simulink model "model_prawego_zbiornika"  (R2023b)
settings: Solver=ode1  StartTime=0.0  StopTime=200  FixedStep=0.02  RelTol=1e-3
undefined symbols (not defined in the file or in its folder): DiscIntNeverNeededParam
libraries: slctrl_adaptive x1, fuzblock x1, slpidlib x1, simulink x1
settings Model: Creator=kerif  LastModifiedBy=kerif
settings ConfigComp: PLC_TargetIDE=codesys35  PLC_MultiTBSigbuilderTimeRange=off  PLC_FoldFBCallOutputVar=off  PLC_RemoveUnusedSSMethodCallArguments=off  PLC_UseCallOutputArgSyntax=off  PLC_EnableUnsignedAndDoubleTypes=off  PLC_EnableUDTSplitting=off  PLC_MaxFieldsInUDT=500  PLC_InlineEnumCastFunction=off

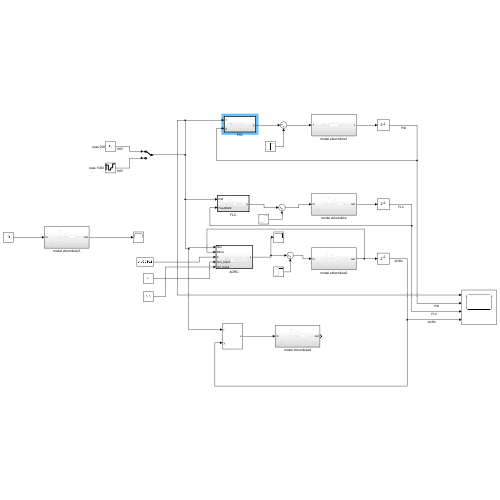
[thumbnail: Simulink's stored preview of the top-level diagram]
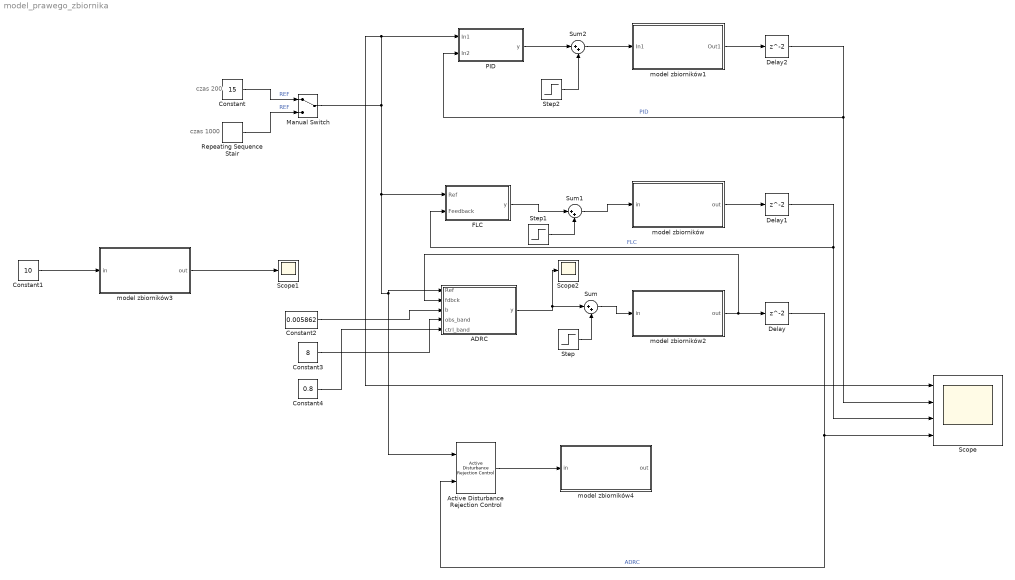
== system model_prawego_zbiornika ==
  note: czas 1000
  note: czas 200
  ADRC : Subsystem  TreatAsAtomicUnit=on
  Active Disturbance Rejection Control : slctrl_adaptive/Active Disturbance Rejection Control  time_domain=discrete-time  Ts=0.02  model_type=first-order  b0=1  wc=3  wo=0.5  x0=0  ulim_checkbox=on  umax=100  umin=0  xhat_checkbox=off
      settings: LibrarySourceBlock=slctrlblks/Adaptive Control/Active Disturbance Rejection Control
  Constant : Constant  Value=15
  Constant1 : Constant  Value=10
  Constant2 : Constant  Value=0.005862
  Constant3 : Constant  Value=8
  Constant4 : Constant  Value=0.8
  Delay : Delay
  Delay1 : Delay
  Delay2 : Delay
  FLC : Subsystem  TreatAsAtomicUnit=on
  Manual Switch : ManualSwitch
  PID : Subsystem  TreatAsAtomicUnit=on
  Repeating Sequence Stair : simulink/Sources/Repeating Sequence Stair  OutValues=[15 5 10 18].'  tsamp=200  OutMin=[]  OutMax=[]  OutDataTypeStr=double  OutputDataTypeScalingMode=double  OutDataType=fixdt(0,8)  ConRadixGroup=Best Precision: Vector-wise  OutScaling=2^-12
  Scope : Scope  NumInputPorts=4
  Scope1 : Scope
  Scope2 : Scope
  Step : Step  Time=100  After=70  SampleTime=0
  Step1 : Step  Time=100  After=70  SampleTime=0
  Step2 : Step  Time=100  After=70  SampleTime=0
  Sum : Sum  Inputs=|++
  Sum1 : Sum  Inputs=|++
  Sum2 : Sum  Inputs=|++
  model zbiorników : Subsystem
  model zbiorników1 : Subsystem
  model zbiorników2 : Subsystem
  model zbiorników3 : Subsystem
  model zbiorników4 : Subsystem
  wires:
  model zbiorników1/1(Out1) -> Delay2/1
  model zbiorników/1(out) -> Delay1/1
  Constant/1 -> Manual Switch/1  "REF"
  Repeating Sequence Stair/1 -> Manual Switch/2  "REF"
  Manual Switch/1 -> Active Disturbance Rejection Control/1, ADRC/1(Ref), FLC/1(Ref), PID/1(In1), Scope/1
  model zbiorników2/1(out) -> Delay/1, ADRC/2(fdbck)
  Constant1/1 -> model zbiorników3/1(in)
  model zbiorników3/1(out) -> Scope1/1
  Active Disturbance Rejection Control/1 -> model zbiorników4/1(in)
  Delay/1 -> Active Disturbance Rejection Control/2, Scope/4  "ADRC"
  Delay1/1 -> Scope/3, FLC/2(Feedback)  "FLC"
  Delay2/1 -> Scope/2, PID/2(In2)  "PID"
  ADRC/1(y) -> Sum/1, Scope2/1
  Sum/1 -> model zbiorników2/1(in)
  Step/1 -> Sum/2
  Step2/1 -> Sum2/2
  PID/1(y) -> Sum2/1
  Sum2/1 -> model zbiorników1/1(In1)
  Step1/1 -> Sum1/2
  FLC/1(y) -> Sum1/1
  Sum1/1 -> model zbiorników/1(in)
  Constant2/1 -> ADRC/3(b)
  Constant3/1 -> ADRC/4(obs_band)
  Constant4/1 -> ADRC/5(ctrl_band)

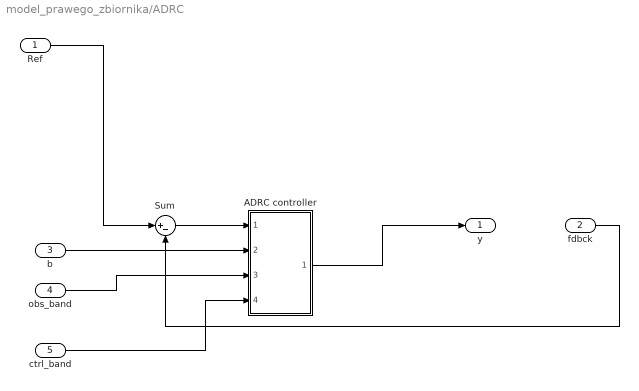
== system model_prawego_zbiornika/ADRC ==
  Ref : Inport
  fdbck : Inport  Port=2
  b : Inport  Port=3
  obs_band : Inport  Port=4
  ctrl_band : Inport  Port=5
  ADRC controller : Subsystem  AncestorBlock=adrc_toolbox_library/ADRC controller  mask(ADRC controller){dynamicsOrder=2, inputGainParameter=0.005862, inputGainSource=External, observerBandwidth=3, observerBandwidthSource=External, controllerBandwidth=0.5, controllerBandwidthSource=External, saturationEnabled=on, UpperLimit=100, LowerLimit=0, deadTimeEnabled=off, deadTime=0.2, observerOutputEnabled=off, observerOutputChoice=Estimated total disturbance}
      mask prompts: dynamicsOrder "Dynamics order (n):"; inputGainParameter "Value:"; inputGainSource "Source:"; observerBandwidth "Value [rad/s]:"; observerBandwidthSource "Source:"; controllerBandwidth "Value [rad/s]:"; controllerBandwidthSource "Source:"; saturationEnabled "Saturation"; UpperLimit "Upper limit (u_max):"; LowerLimit "Lower limit (u_min):"; deadTimeEnabled "Anti-peaking"; deadTime "Controller start time [s] (T_d):"; observerOutputEnabled "Show observer output"; observerOutputChoice "Observer output type"
      mask help: The ADRC controller is a part of the Active Disturbance Rejection Control (ADRC) Toolbox, available at: https://www.mathworks.com/matlabcentral/fileexchange/102249-active-disturbance-rejection-control-adrc-toolbox
      mask init:
      | set_param(gcb,'MaskHideContents','off');
      | set_param(gcb, 'MaskSelfModifiable', 'on');
      | 
      | inputGainSource = get_param(gcb,'inputGainSource');
      | switch(inputGainSource)
      |     case 'Internal'
      |         replace_block([gcb,'/inputGainParameterIn'], 'Inport', 'Ground', 'noprompt');
      |         inputGainParameterType = 'Internal';
      |     case 'External'
      |         replace_block([gcb,'/inputGainParameterIn'], 'Ground', 'Inport', 'noprompt');
      |         inputGainParameterType = 'External';
      | end
      | 
      | observerBandwidthSource = get_param(gcb,'observerBandwidthSource');
      | switch(observerBandwidthSource)
      |     case 'Internal'
      |         replace_block([gcb,'/observerBandwidthIn'], 'Inport', 'Ground', 'noprompt');
      |         inputGainParameterType = 'Internal';
      |     case 'External'
      |         replace_block([gcb,'/observerBandwidthIn'], 'Ground', 'Inport', 'noprompt');
      |         inputGainParameterType = 'External';
      | end
      | 
      | controllerBandwidthSource = get_param(gcb,'controllerBandwidthSource');
      | switch(controllerBandwidthSource)
      |     case 'Internal'
      |         replace_block([gcb,'/controllerBandwidthIn'], 'Inport', 'Ground', 'noprompt');
      |         inputGainParameterType = 'Internal';
      |     case 'External'
      |         replace_block([gcb,'/controllerBandwidthIn'], 'Ground', 'Inport', 'noprompt');
      |         inputGainParameterType = 'External';
      | end
      | 
      | observerOutputEnabled = get_param(gcb,'observerOutputEnabled');
      | switch(observerOutputEnabled)
      |     case 'off'
      |         replace_block([gcb,'/selectedObserverOutput'], 'Outport', 'Terminator', 'noprompt');
      |     case 'on'
      |         replace_block([gcb,'/selectedObserverOutput'], 'Terminator', 'Outport', 'noprompt');
      | end
      mask Help:
      | The ADRC controller is a single, drag-and-drop, Simulink function block that encapsulates a specific continuous-time error-based active disturbance rejection control (ADRC) algorithm. For simplicity and compactness, the ADRC controller is developed as a single-input (feedback error signal), single-output (control signal) block, which can be used as a powerful alternative to the conventional PID controller.
      | 
      | The design parameters of the implemented ADRC algorithm can be easily changed using the provided graphical user interface (GUI). The GUI also allows to activate two practical functionalities, namely: saturation of the control signal and anti-peaking mechanism.
      | 
      | The ADRC controller is a part of the Active Disturbance Rejection Control (ADRC) Toolbox. The goal of the Active Disturbance Rejection Control (ADRC) Toolbox is to provide an intuitive control solution for Simulink, allowing the implementation of ADRC algorithm in simulations/experiments quickly and with low effort.
      | 
      | A pre-print containing detailed information about the developed ADRC Toolbox can be found here:
      | https://arxiv.org/abs/2112.01614
      | 
      | Code contributors: Krzysztof Lakomy, Rafal Madonski, Jacek Michalski, Wojciech Giernacki
      | 
      | Contact: adrc.toolbox@gmail.com
      | 
      | ADRC Toolbox at MathWorks File Exchange:
      | https://www.mathworks.com/matlabcentral/fileexchange/102249-active-disturbance-rejection-control-adrc-toolbox
      mask TypeOptions dynamicsOrder: Linear extended state observer/dynamicsOrder | State feedback robust controller/dynamicsOrder
      mask TypeOptions inputGainParameter: Linear extended state observer/inputGainParameter | State feedback robust controller/inputGainParameter
      mask TypeOptions inputGainSource: Internal | External
      mask Callback inputGainSource:
      | inputGainSource = get_param(gcb,'inputGainSource');
      | 
      | nameList = get_param(gcb, 'MaskNames');
      | enableList = get_param(gcb, 'MaskEnables');
      | inputGainParameterIndex = find(strcmp(nameList, 'inputGainParameter'));
      | 
      | switch(inputGainSource)
      |     case 'Internal'
      |         enableList{inputGainParameterIndex} = 'on';
      |     case 'External'
      |         enableList{inputGainParameterIndex} = 'off';
      | end
      | 
      | set_param(gcb,'MaskEnables',enableList);
      mask TypeOptions observerBandwidth: Linear extended state observer/observerBandwidth
      mask TypeOptions observerBandwidthSource: Internal | External
      mask Callback observerBandwidthSource:
      | observerBandwidthSource = get_param(gcb,'observerBandwidthSource');
      | 
      | nameList = get_param(gcb, 'MaskNames');
      | enableList = get_param(gcb, 'MaskEnables');
      | observerBandwidthIndex = find(strcmp(nameList, 'observerBandwidth'));
      | 
      | switch(observerBandwidthSource)
      |     case 'Internal'
      |         enableList{observerBandwidthIndex} = 'on';
      |     case 'External'
      |         enableList{observerBandwidthIndex} = 'off';
      | end
      | 
      | set_param(gcb,'MaskEnables',enableList);
      mask TypeOptions controllerBandwidth: State feedback robust controller/controllerBandwidth
      mask TypeOptions controllerBandwidthSource: Internal | External
      mask Callback controllerBandwidthSource:
      | controllerBandwidthSource = get_param(gcb,'controllerBandwidthSource');
      | 
      | nameList = get_param(gcb, 'MaskNames');
      | enableList = get_param(gcb, 'MaskEnables');
      | controllerBandwidthIndex = find(strcmp(nameList, 'controllerBandwidth'));
      | 
      | switch(controllerBandwidthSource)
      |     case 'Internal'
      |         enableList{controllerBandwidthIndex} = 'on';
      |     case 'External'
      |         enableList{controllerBandwidthIndex} = 'off';
      | end
      | 
      | set_param(gcb,'MaskEnables',enableList);
      mask TypeOptions saturationEnabled: State feedback robust controller/saturationEnabled
      mask Callback saturationEnabled:
      | saturationEnabled = get_param(gcb, 'saturationEnabled');
      | 
      | nameList = get_param(gcb, 'MaskNames');
      | enableList = get_param(gcb, 'MaskEnables');
      | upperLimitIndex = find(strcmp(nameList, 'UpperLimit'));
      | lowerLimitIndex = find(strcmp(nameList, 'LowerLimit'));
      | 
      | switch(saturationEnabled)
      |     case 'on'
      |         enableList{upperLimitIndex} = 'on';
      |         enableList{lowerLimitIndex} = 'on';
      |     case 'off'
      |         enableList{upperLimitIndex} = 'off';
      |         enableList{lowerLimitIndex} = 'off';
      | end
      | 
      | set_param(gcb,'MaskEnables',enableList);
      mask TypeOptions UpperLimit: State feedback robust controller/UpperLimit
      mask TypeOptions LowerLimit: State feedback robust controller/LowerLimit
      mask TypeOptions deadTimeEnabled: State feedback robust controller/deadTimeEnabled
      mask Callback deadTimeEnabled:
      | deadTimeEnabled = get_param(gcb,'deadTimeEnabled');
      | 
      | nameList = get_param(gcb, 'MaskNames');
      | enableList = get_param(gcb, 'MaskEnables');
      | deadTimeIndex = find(strcmp(nameList, 'deadTime'));
      | 
      | switch(deadTimeEnabled)
      |     case 'on'
      |         enableList{deadTimeIndex} = 'on';
      |     case 'off'
      |         enableList{deadTimeIndex} = 'off';
      | end
      | 
      | set_param(gcb,'MaskEnables',enableList);
      mask TypeOptions deadTime: State feedback robust controller/Time
      mask Callback observerOutputEnabled:
      | observerOutputEnabled = get_param(gcb,'observerOutputEnabled');
      | 
      | nameList = get_param(gcb, 'MaskNames');
      | enableList = get_param(gcb, 'MaskEnables');
      | observerOutputChoiceIndex = find(strcmp(nameList, 'observerOutputChoice'));
      | 
      | switch(observerOutputEnabled)
      |     case 'on'
      |         enableList{observerOutputChoiceIndex} = 'on';
      |     case 'off'
      |         enableList{observerOutputChoiceIndex} = 'off';
      | end
      | 
      | set_param(gcb,'MaskEnables',enableList);
      mask TypeOptions observerOutputChoice: Observer output/observerOutputChoice
      mask DialogControl DescGroupVar Prompt: Active Disturbance Rejection Controller (ADRC)
      mask DialogControl DescTextVar Prompt: This block implements a linear continuous-time error-based Active Disturbance Rejection Controller (ADRC). The default form of this controller calculates the control signal (block output) based on the control feedback error (block input).
      mask DialogControl ParameterGroupVar Prompt: Control system parameters and functionalities
      mask DialogControl Container5 Prompt: Parameters
      mask DialogControl Container10 Prompt: Input gain (hat_b):
      mask DialogControl Container11 Prompt: Observer bandwidth (omega_o):
      mask DialogControl Container12 Prompt: Controller bandwidth (omega_c):
      mask DialogControl Container4 Prompt: Saturation
      mask DialogControl Control3 Prompt: Saturation functionality limits the boundary values of the control signal, allowing to adjust the output of the ADRC controller block to the physical limitations of the controlled system.
      mask DialogControl Container8 Prompt: Anti-peaking
      mask DialogControl Control4 Prompt: Anti-peaking functionality is obtained by delaying the controller start by an user-defined time value (in seconds), allowing the observer transient state to pass.
      mask DialogControl Container21 Prompt: Observer output
      mask DialogControl Control5 Prompt: Observer output allows showing selected signals estimated by the built-in observer.
      mask Display:
      | inputGainSource = get_param(gcb,'inputGainSource');
      | observerBandwidthSource = get_param(gcb,'observerBandwidthSource');
      | controllerBandwidthSource = get_param(gcb,'controllerBandwidthSource');
      | observerOutputEnabled = get_param(gcb,'observerOutputEnabled');
      | observerOutputChoice = get_param(gcb, 'observerOutputChoice');
      | 
      | disp('ADRC');
      | 
      | switch inputGainSource
      |     case 'Internal'
      |     case 'External'
      |         port_label('input',1,'e');
      |         port_label('input',2,'hat_b');
      | end
      | 
      | switch observerBandwidthSource
      |     case 'Internal'
      |     case 'External'
      |         port_label('input',1,'e');
      |         if(strcmp(inputGainSource,'External'))
      |             port_label('input',3,'omega_o');
      |         else
      |             port_label('input',2,'omega_o');
      |         end
      | end
      | 
      | switch controllerBandwidthSource
      |     case 'Internal'
      |     case 'External'
      |         port_label('input',1,'e');
      |         if(strcmp(inputGainSource,'External') && strcmp(observerBandwidthSource,'External'))
      |             port_label('input',4,'omega_c');
      |         elseif(xor(strcmp(inputGainSource,'External'), strcmp(observerBandwidthSource,'External')))
      |             port_label('input',3,'omega_c');
      |         else
      |             port_label('input',2,'omega_c');
      |         end
      | end
      | 
      | switch observerOutputEnabled
      |     case 'off'
      |     case 'on'
      |         port_label('output',1,'u');
      |         if(strcmp(observerOutputChoice,'Estimated total disturbance'))
      |             port_label('output',2,'hat_f');
      |         elseif(strcmp(observerOutputChoice,'Estimated extended state'))
      |             port_label('output',2,'hat_z');
      |         elseif(strcmp(observerOutputChoice,'Estimated control error'))
      |             port_label('output',2,'hat_e');
      |         end
      | end
  Sum : Sum  Inputs=|+-
  y : Outport
  wires:
  Sum/1 -> ADRC controller/1(controlError)
  fdbck/1 -> Sum/2
  ADRC controller/1(controlSignal) -> y/1
  Ref/1 -> Sum/1
  b/1 -> ADRC controller/2(inputGainParameterIn)
  obs_band/1 -> ADRC controller/3(observerBandwidthIn)
  ctrl_band/1 -> ADRC controller/4(controllerBandwidthIn)

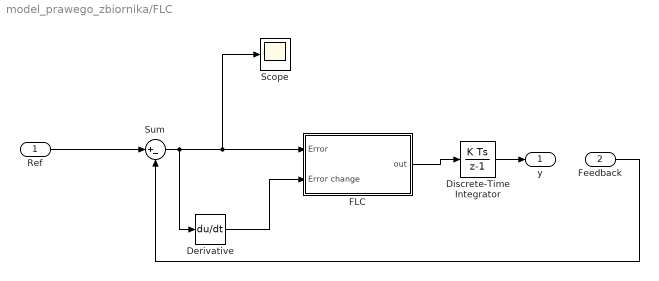
== system model_prawego_zbiornika/FLC ==
  Ref : Inport
  Feedback : Inport  Port=2
  Derivative : Derivative
  Discrete-Time Integrator : DiscreteIntegrator  SampleTime=0.2  ICPrevOutput=DiscIntNeverNeededParam  ICPrevScaledInput=DiscIntNeverNeededParam
  FLC : Subsystem  TreatAsAtomicUnit=on  SystemSampleTime=0.02
  Scope : Scope
  Sum : Sum  Inputs=|+-
  y : Outport
  wires:
  Feedback/1 -> Sum/2
  Ref/1 -> Sum/1
  Sum/1 -> Derivative/1, Scope/1, FLC/1(Error)
  Derivative/1 -> FLC/2(Error change)
  FLC/1(out) -> Discrete-Time Integrator/1
  Discrete-Time Integrator/1 -> y/1

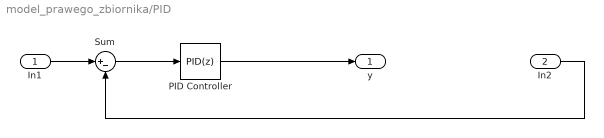
== system model_prawego_zbiornika/PID ==
  In1 : Inport
  In2 : Inport  Port=2
  PID Controller : slpidlib/PID Controller  Controller=PID  Form=Parallel  TimeDomain=Discrete-time  UseExternalTs=off  SampleTime=0.02  IntegratorMethod=Forward Euler  FilterMethod=Forward Euler  ControllerParametersSource=internal  P=9.43464394220786  I=0.67318018767203  UseKiTs=off  D=21.7349674504552  N=0.537912666068036  UseFilter=on  TunerSelectOption=Transfer Function Based (PID Tuner App)  ZeroCross=off  InitialConditionSource=internal  InitialConditionForIntegrator=0  InitialConditionForFilter=0  DifferentiatorICPrevScaledInput=0  ExternalReset=none  TrackingMode=off  Kt=1  LimitOutput=on  SatLimitsSource=internal  UpperSaturationLimit=100  LowerSaturationLimit=0  LinearizeAsGain=on  AntiWindupMode=none  Kb=1  LimitIntegrator=off  UpperIntegratorSaturationLimit=inf  LowerIntegratorSaturationLimit=-inf  POutMin=[]  POutMax=[]  IOutMin=[]  IOutMax=[]  DOutMin=[]  DOutMax=[]  NOutMin=[]  NOutMax=[]  SumOutMin=[]  SumOutMax=[]  SaturationOutMin=[]  SaturationOutMax=[]  PParamMin=[]  PParamMax=[]  IParamMin=[]  IParamMax=[]  DParamMin=[]  DParamMax=[]  NParamMin=[]  NParamMax=[]  KbParamMin=[]  KbParamMax=[]  KtParamMin=[]  KtParamMax=[]  KbOutMin=[]  KbOutMax=[]  KtOutMin=[]  KtOutMax=[]  IntegratorOutMin=[]  IntegratorOutMax=[]  FilterOutMin=[]  FilterOutMax=[]  SumI1OutMin=[]  SumI1OutMax=[]  SumI2OutMin=[]  SumI2OutMax=[]  SumI3OutMin=[]  SumI3OutMax=[]  SumI4OutMin=[]  SumI4OutMax=[]  SumDOutMin=[]  SumDOutMax=[]  DifferentiatorOutMin=[]  DifferentiatorOutMax=[]  FilterDiffOutCoefMin=[]  FilterDiffOutCoefMax=[]  ReciprocalOutMin=[]  ReciprocalOutMax=[]  SumDenOutMin=[]  SumDenOutMax=[]  SumNumOutMin=[]  SumNumOutMax=[]  DivideOutMin=[]  DivideOutMax=[]  UdiffTsProdOutMin=[]  UdiffTsProdOutMax=[]  NTsProdOutMin=[]  NTsProdOutMax=[]  UintegralTsProdOutMin=[]  UintegralTsProdOutMax=[]  UngainTsProdOutMin=[]  UngainTsProdOutMax=[]  ClampingZeroOutDataTypeStr=Inherit: Inherit via back propagation  ClampingZeroOutMin=[]  ClampingZeroOutMax=[]  FilterDenConstantOutDataTypeStr=Inherit: Inherit via back propagation  FilterDenConstantOutMin=[]  FilterDenConstantOutMax=[]  PCopyOutDataTypeStr=Inherit: Inherit via back propagation  PCopyOutMin=[]  PCopyOutMax=[]  NCopyOutDataTypeStr=Inherit: Inherit via back propagation  NCopyOutMin=[]  NCopyOutMax=[]  IntegratorContinuousStateAttributes=''  IntegratorStateMustResolveToSignalObject=off  IntegratorRTWStateStorageClass=Auto  FilterContinuousStateAttributes=''  FilterStateMustResolveToSignalObject=off  FilterRTWStateStorageClass=Auto  ParallelPVariant=InternalParameters  IdealPVariant=Disabled  IVariant=InternalParameters  DVariant=InternalParameters  IntegratorVariant=Discrete  SatVariant=Enabled  AWVariant=Passthrough  PCopyVariant=Disabled  TRVariant=Disabled  FdbkBlocksVariant=Forward  IdealPFdbkVariant=Disabled  SatFdbkVariant=Disabled  DerivativeFilterVariant=ForwardEulerFilter  NVariant=InternalParameters  NCopyVariant=Disabled  FilterICVariant=InternalICsFilter  IntegratorICVariant=InternalICs  ExternalResetVariant=Disabled  TRSumVariant=Passthrough  SumFdbkVariant=Disabled  SumVariant=Sum_PID  TsampFilterVariant=InternalTs  TsampNgainVariant=Passthrough  TsampIntegralVariant=Disabled_SignalSpec  ExternalSaturationOutDataTypeStr=Inherit: Same as second input
  Sum : Sum  Inputs=|+-
  y : Outport
  wires:
  In1/1 -> Sum/1
  In2/1 -> Sum/2
  PID Controller/1 -> y/1
  Sum/1 -> PID Controller/1

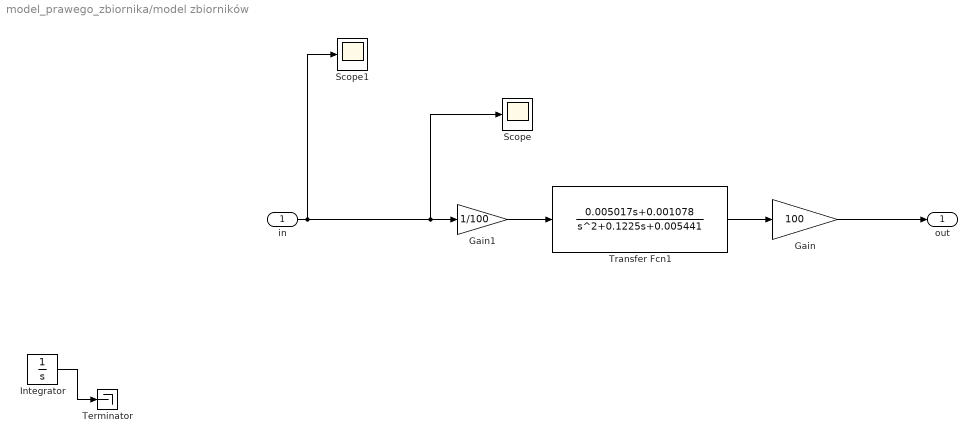
== system model_prawego_zbiornika/model zbiorników ==
  in : Inport
  Gain : Gain  Gain=100
  Gain1 : Gain  Gain=1/100
  Integrator : Integrator  LimitOutput=on  UpperSaturationLimit=100  LowerSaturationLimit=-100
  Scope : Scope
  Scope1 : Scope
  Terminator : Terminator
  Transfer Fcn1 : TransferFcn  Numerator=[0.005017 0.001078]  Denominator=[1 0.1225 0.005441]
  out : Outport
  wires:
  Gain1/1 -> Transfer Fcn1/1
  Transfer Fcn1/1 -> Gain/1
  Gain/1 -> out/1
  Integrator/1 -> Terminator/1
  in/1 -> Scope/1, Gain1/1, Scope1/1

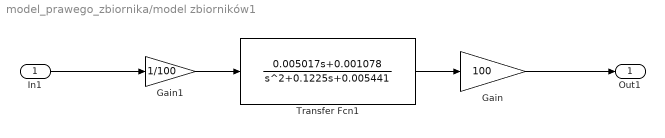
== system model_prawego_zbiornika/model zbiorników1 ==
  In1 : Inport
  Gain : Gain  Gain=100
  Gain1 : Gain  Gain=1/100
  Transfer Fcn1 : TransferFcn  Numerator=[0.005017 0.001078]  Denominator=[1 0.1225 0.005441]
  Out1 : Outport
  wires:
  Gain1/1 -> Transfer Fcn1/1
  Transfer Fcn1/1 -> Gain/1
  In1/1 -> Gain1/1
  Gain/1 -> Out1/1

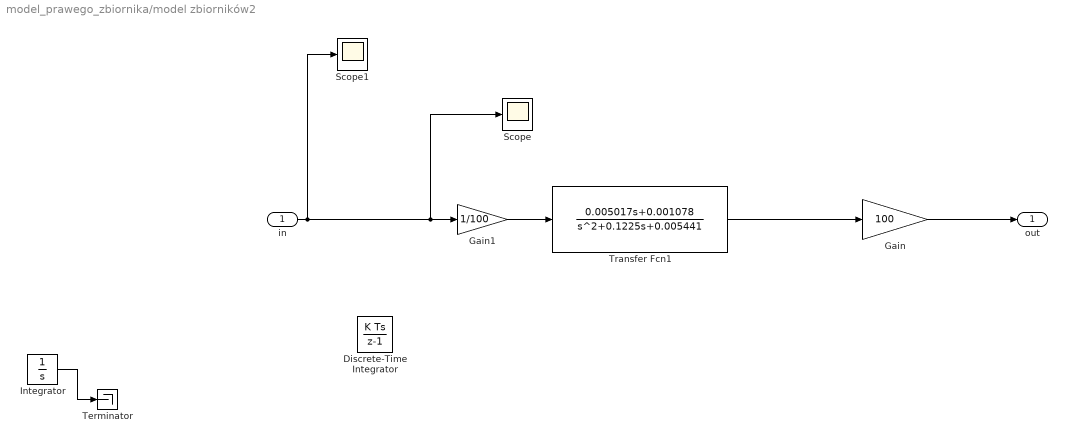
== system model_prawego_zbiornika/model zbiorników2 ==
  in : Inport
  Discrete-Time Integrator : DiscreteIntegrator  SampleTime=0.2  ICPrevOutput=DiscIntNeverNeededParam  ICPrevScaledInput=DiscIntNeverNeededParam
  Gain : Gain  Gain=100
  Gain1 : Gain  Gain=1/100
  Integrator : Integrator  LimitOutput=on  UpperSaturationLimit=100  LowerSaturationLimit=-100
  Scope : Scope
  Scope1 : Scope
  Terminator : Terminator
  Transfer Fcn1 : TransferFcn  Numerator=[0.005017 0.001078]  Denominator=[1 0.1225 0.005441]
  out : Outport
  wires:
  Gain1/1 -> Transfer Fcn1/1
  Transfer Fcn1/1 -> Gain/1
  Gain/1 -> out/1
  in/1 -> Scope/1, Gain1/1, Scope1/1
  Integrator/1 -> Terminator/1

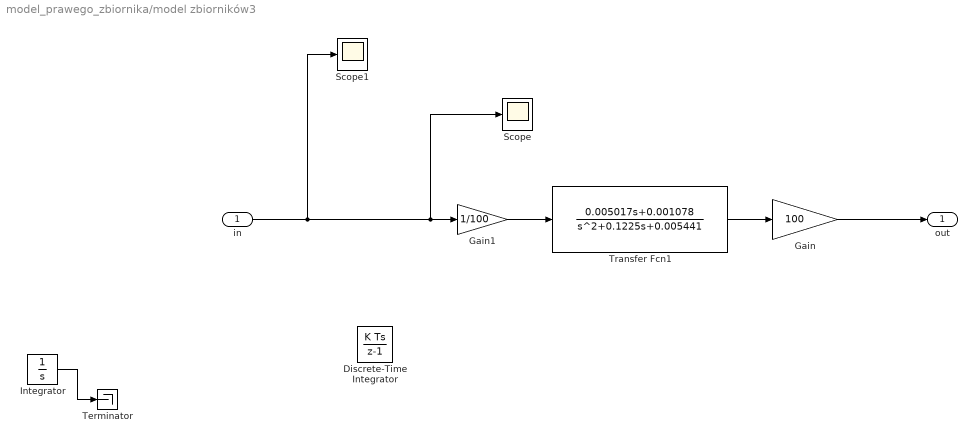
== system model_prawego_zbiornika/model zbiorników3 ==
  in : Inport
  Discrete-Time Integrator : DiscreteIntegrator  SampleTime=0.2  ICPrevOutput=DiscIntNeverNeededParam  ICPrevScaledInput=DiscIntNeverNeededParam
  Gain : Gain  Gain=100
  Gain1 : Gain  Gain=1/100
  Integrator : Integrator  LimitOutput=on  UpperSaturationLimit=100  LowerSaturationLimit=-100
  Scope : Scope
  Scope1 : Scope
  Terminator : Terminator
  Transfer Fcn1 : TransferFcn  Numerator=[0.005017 0.001078]  Denominator=[1 0.1225 0.005441]
  out : Outport
  wires:
  Gain1/1 -> Transfer Fcn1/1
  Transfer Fcn1/1 -> Gain/1
  Gain/1 -> out/1
  in/1 -> Scope/1, Gain1/1, Scope1/1
  Integrator/1 -> Terminator/1

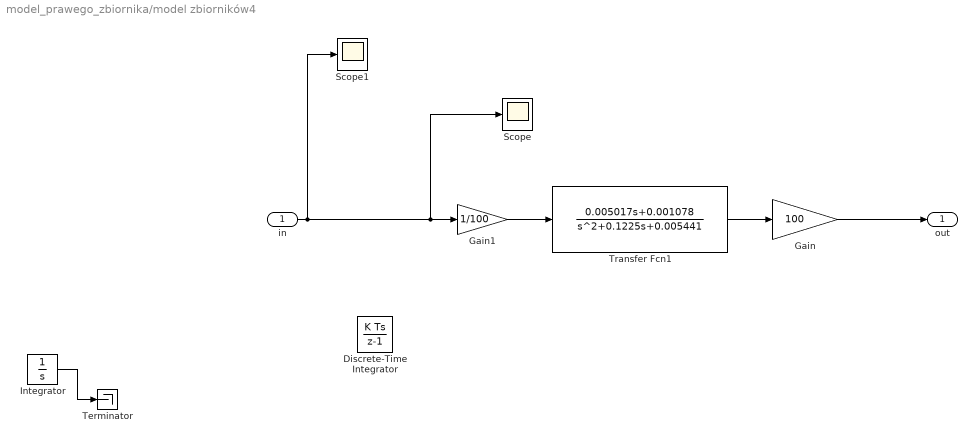
== system model_prawego_zbiornika/model zbiorników4 ==
  in : Inport
  Discrete-Time Integrator : DiscreteIntegrator  SampleTime=0.2  ICPrevOutput=DiscIntNeverNeededParam  ICPrevScaledInput=DiscIntNeverNeededParam
  Gain : Gain  Gain=100
  Gain1 : Gain  Gain=1/100
  Integrator : Integrator  LimitOutput=on  UpperSaturationLimit=100  LowerSaturationLimit=-100
  Scope : Scope
  Scope1 : Scope
  Terminator : Terminator
  Transfer Fcn1 : TransferFcn  Numerator=[0.005017 0.001078]  Denominator=[1 0.1225 0.005441]
  out : Outport
  wires:
  Gain1/1 -> Transfer Fcn1/1
  Transfer Fcn1/1 -> Gain/1
  Gain/1 -> out/1
  in/1 -> Scope/1, Gain1/1, Scope1/1
  Integrator/1 -> Terminator/1

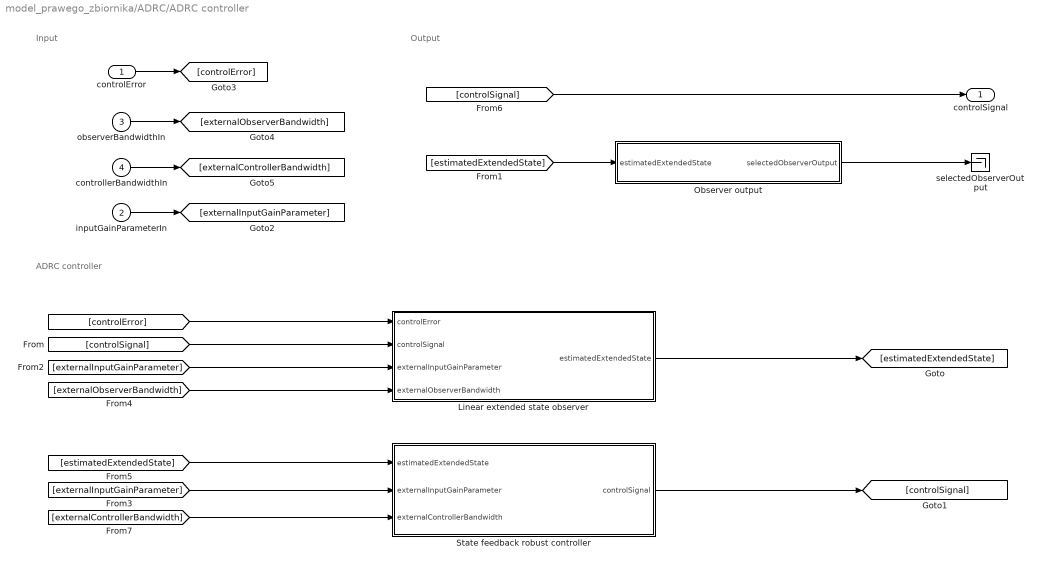
== system model_prawego_zbiornika/ADRC/ADRC controller ==
  note: Input
  note: Output
  note: ADRC controller
  controlError : Inport
  inputGainParameterIn : Inport  Port=2
  observerBandwidthIn : Inport  Port=3
  controllerBandwidthIn : Inport  Port=4
  Linear extended state observer : Subsystem  mask{InitialCondition=zeros(dynamicsOrder+1,1), dynamicsOrder=dynamicsOrder, observerBandwidth=observerBandwidth, inputGainParameter=inputGainParameter}
      mask prompts: InitialCondition "Integrator initial conditions:"; dynamicsOrder "Dynamics order:"; observerBandwidth "Observer bandwidth:"; inputGainParameter "Input gain parameter:"
      mask TypeOptions InitialCondition: Integrator/InitialCondition
      mask TypeOptions dynamicsOrder: Linear extended state observer/dynamicsOrder
      mask TypeOptions observerBandwidth: Linear extended state observer/observerBandwidth
      mask TypeOptions inputGainParameter: Linear extended state observer/inputGainParameter
  Observer output : Subsystem  Variant=on  VariantControlMode=label  LabelModeActiveChoice=estimated_total_disturbance  mask{observerOutputChoice=Estimated total disturbance}
      mask prompts: observerOutputChoice "Observer output:"
      mask TypeOptions observerOutputChoice: Estimated total disturbance | Estimated extended state | Estimated control error
      mask Callback observerOutputChoice:
      | observerOutputChoice = get_param(gcb,'observerOutputChoice');
      | if strcmp(observerOutputChoice,'Estimated total disturbance')
      |     set_param(gcb, 'LabelModeActiveChoice', 'estimated_total_disturbance');
      | elseif strcmp(observerOutputChoice, 'Estimated extended state')
      |     set_param(gcb, 'LabelModeActiveChoice', 'estimated_extended_state')
      | elseif strcmp(observerOutputChoice, 'Estimated control error')
      |     set_param(gcb, 'LabelModeActiveChoice', 'estimated_control_error')
      | else
      |     set_param(gcb, 'LabelModeActiveChoice', 'estimated_total_disturbance');
      | end
  State feedback robust controller : Subsystem  mask{dynamicsOrder=dynamicsOrder, inputGainParameter=inputGainParameter, controllerBandwidth=controllerBandwidth, saturationEnabled=on, UpperLimit=UpperLimit, LowerLimit=LowerLimit, deadTimeEnabled=off, Time=deadTime}
      mask prompts: dynamicsOrder "Dynamics order:"; inputGainParameter "Input gain parameter:"; controllerBandwidth "Controller bandwidth:"; saturationEnabled "Output saturation"; UpperLimit "Simulink:blkprm_prompts:SaturateUpLim"; LowerLimit "Simulink:blkprm_prompts:SaturateLowLim"; deadTimeEnabled "Dead time enabled"; Time "Dead time:"
      mask TypeOptions dynamicsOrder: Extended state feedback robust controller/dynamicsOrder
      mask TypeOptions inputGainParameter: Extended state feedback robust controller/inputGainParameter
      mask TypeOptions controllerBandwidth: Extended state feedback robust controller/controllerBandwidth
      mask TypeOptions saturationEnabled: Saturation/saturationEnabled
      mask TypeOptions UpperLimit: Saturation/UpperLimit
      mask TypeOptions LowerLimit: Saturation/LowerLimit
      mask TypeOptions deadTimeEnabled: Dead time/deadTimeEnabled
      mask TypeOptions Time: Dead time/Time
      mask DialogControl UpperLimit Prompt: Upper limit:
      mask DialogControl LowerLimit Prompt: Lower limit:
  selectedObserverOutput : Terminator
  controlSignal : Outport
  wires:
  Observer output/1(selectedObserverOutput) -> selectedObserverOutput/1
  [estimatedExtendedState] -> Observer output/1(estimatedExtendedState)
  [externalControllerBandwidth] -> State feedback robust controller/3(externalControllerBandwidth)
  controllerBandwidthIn/1 -> [externalControllerBandwidth]
  [externalObserverBandwidth] -> Linear extended state observer/4(externalObserverBandwidth)
  observerBandwidthIn/1 -> [externalObserverBandwidth]
  State feedback robust controller/1(controlSignal) -> [controlSignal]
  [externalInputGainParameter] -> State feedback robust controller/2(externalInputGainParameter)
  [externalInputGainParameter] -> Linear extended state observer/3(externalInputGainParameter)
  inputGainParameterIn/1 -> [externalInputGainParameter]
  [estimatedExtendedState] -> State feedback robust controller/1(estimatedExtendedState)
  Linear extended state observer/1(estimatedExtendedState) -> [estimatedExtendedState]
  controlError/1 -> [controlError]
  [controlSignal] -> Linear extended state observer/2(controlSignal)
  [controlError] -> Linear extended state observer/1(controlError)
  [controlSignal] -> controlSignal/1

== system model_prawego_zbiornika/FLC/FLC ==
  Error : Inport
  Error change : Inport  Port=2
  Fuzzy Logic Controller : fuzblock/Fuzzy Logic  Controller  FIS=FLC_PD_1  OutputSampleNumber=101  DataType=double  FuzzifiedInputs=off  RuleFiringStrengths=off  RuleOutputs=off  AggregatedOutputs=off  SimulateUsing=Interpreted execution  OutOfRangeInputValueMessage=warning  NoRuleFiredMessage=warning  EmptyOutputFuzzySetMessage=warning
  Mux : Mux  Inputs=2
  out : Outport
  wires:
  Mux/1 -> Fuzzy Logic Controller/1
  Fuzzy Logic Controller/1 -> out/1
  Error/1 -> Mux/1
  Error change/1 -> Mux/2

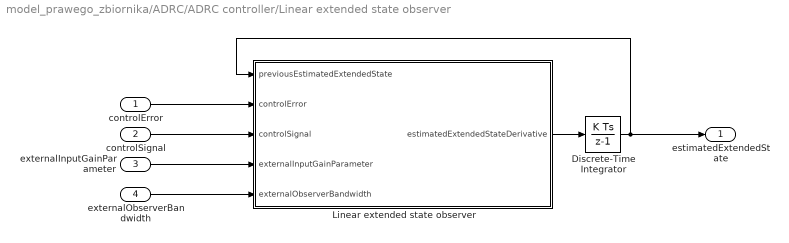
== system model_prawego_zbiornika/ADRC/ADRC controller/Linear extended state observer ==
  controlError : Inport
  controlSignal : Inport  Port=2
  externalInputGainParameter : Inport  Port=3  PortDimensions=1
  externalObserverBandwidth : Inport  Port=4  PortDimensions=1
  Discrete-Time Integrator : DiscreteIntegrator  SampleTime=-1  ICPrevOutput=DiscIntNeverNeededParam  ICPrevScaledInput=DiscIntNeverNeededParam
  Linear extended state observer : MATLAB Function  TreatAsAtomicUnit=on  mask{dynamicsOrder=dynamicsOrder, observerBandwidth=observerBandwidth, inputGainParameter=inputGainParameter}
      mask prompts: dynamicsOrder "Dynamics order:"; observerBandwidth "Observer bandwidth:"; inputGainParameter "Input gain parameter:"
  estimatedExtendedState : Outport
  wires:
  externalObserverBandwidth/1 -> Linear extended state observer/5(externalObserverBandwidth)
  Discrete-Time Integrator/1 -> estimatedExtendedState/1, Linear extended state observer/1(previousEstimatedExtendedState)
  controlSignal/1 -> Linear extended state observer/3(controlSignal)
  externalInputGainParameter/1 -> Linear extended state observer/4(externalInputGainParameter)
  Linear extended state observer/1(estimatedExtendedStateDerivative) -> Discrete-Time Integrator/1
  controlError/1 -> Linear extended state observer/2(controlError)

== system model_prawego_zbiornika/ADRC/ADRC controller/Observer output ==
  estimatedExtendedState : Inport
  Only estimated control error : Subsystem  VariantControl=estimated_control_error
  Only estimated total disturbance : Subsystem  VariantControl=estimated_total_disturbance
  Whole estimated extended state : Subsystem  VariantControl=estimated_extended_state
  selectedObserverOutput : Outport

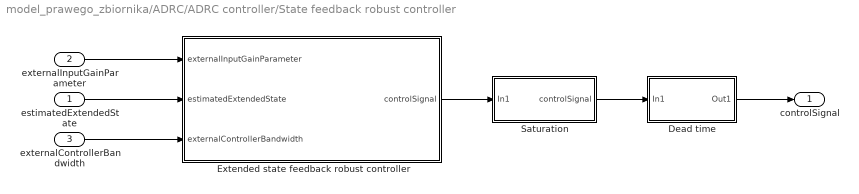
== system model_prawego_zbiornika/ADRC/ADRC controller/State feedback robust controller ==
  estimatedExtendedState : Inport  PortDimensions=dynamicsOrder+1
  externalInputGainParameter : Inport  Port=2  PortDimensions=1  SampleTime=1
  externalControllerBandwidth : Inport  Port=3  PortDimensions=1
  Dead time : Subsystem  Variant=on  VariantControlMode=label  LabelModeActiveChoice=dead_time_off  mask{deadTimeEnabled=off, Time=Time}
      mask prompts: deadTimeEnabled "Dead time enabled"; Time "Dead time:"
      mask Callback deadTimeEnabled:
      | deadTimeChoice = get_param(gcb,'deadTimeEnabled');
      | if strcmp(deadTimeChoice,'off')
      |     set_param(gcb, 'LabelModeActiveChoice', 'dead_time_off');
      | else
      |     set_param(gcb, 'LabelModeActiveChoice', 'dead_time_on');
      | end
      mask TypeOptions Time: Dead time on/Step/Time
  Extended state feedback robust controller : MATLAB Function  TreatAsAtomicUnit=on  mask{dynamicsOrder=dynamicsOrder, inputGainParameter=inputGainParameter, controllerBandwidth=controllerBandwidth}
      mask prompts: dynamicsOrder "Dynamics order:"; inputGainParameter "Input gain parameter:"; controllerBandwidth "Controller bandwidth:"
  Saturation : Subsystem  Variant=on  VariantControlMode=label  LabelModeActiveChoice=saturation_on  mask{saturationEnabled=on, UpperLimit=UpperLimit, LowerLimit=LowerLimit}
      mask prompts: saturationEnabled "Output saturation"; UpperLimit "Simulink:blkprm_prompts:SaturateUpLim"; LowerLimit "Simulink:blkprm_prompts:SaturateLowLim"
      mask Callback saturationEnabled:
      | saturationChoice = get_param(gcb,'saturationEnabled');
      | if strcmp(saturationChoice,'off')
      |     set_param(gcb, 'LabelModeActiveChoice', 'saturation_off');
      | else
      |     set_param(gcb, 'LabelModeActiveChoice', 'saturation_on');
      | end
      mask TypeOptions UpperLimit: Saturation on/Saturation/UpperLimit
      mask TypeOptions LowerLimit: Saturation on/Saturation/LowerLimit
      mask DialogControl UpperLimit Prompt: Upper limit:
      mask DialogControl LowerLimit Prompt: Lower limit:
  controlSignal : Outport
  wires:
  Dead time/1(Out1) -> controlSignal/1
  Saturation/1(controlSignal) -> Dead time/1(In1)
  externalControllerBandwidth/1 -> Extended state feedback robust controller/3(externalControllerBandwidth)
  Extended state feedback robust controller/1(controlSignal) -> Saturation/1(In1)
  externalInputGainParameter/1 -> Extended state feedback robust controller/1(externalInputGainParameter)
  estimatedExtendedState/1 -> Extended state feedback robust controller/2(estimatedExtendedState)

== system model_prawego_zbiornika/ADRC/ADRC controller/Observer output/Only estimated control error ==
  estimatedExtendedState : Inport
  First element of estimated extended state : MATLAB Function  TreatAsAtomicUnit=on  VariantControl=Choice
  selectedObserverOutput : Outport
  wires:
  First element of estimated extended state/1(y) -> selectedObserverOutput/1
  estimatedExtendedState/1 -> First element of estimated extended state/1(u)

== system model_prawego_zbiornika/ADRC/ADRC controller/Observer output/Only estimated total disturbance ==
  estimatedExtendedState : Inport
  Last element of estimated extended state : MATLAB Function  TreatAsAtomicUnit=on
  selectedObserverOutput : Outport
  wires:
  Last element of estimated extended state/1(y) -> selectedObserverOutput/1
  estimatedExtendedState/1 -> Last element of estimated extended state/1(u)

== system model_prawego_zbiornika/ADRC/ADRC controller/Observer output/Whole estimated extended state ==
  estimatedExtendedState : Inport
  selectedObserverOutput : Outport
  wires:
  estimatedExtendedState/1 -> selectedObserverOutput/1

== system model_prawego_zbiornika/ADRC/ADRC controller/State feedback robust controller/Dead time ==
  In1 : Inport
  Dead time off : Subsystem  VariantControl=dead_time_off
  Dead time on : Subsystem  VariantControl=dead_time_on
  Out1 : Outport

== system model_prawego_zbiornika/ADRC/ADRC controller/State feedback robust controller/Saturation ==
  In1 : Inport
  Saturation off : Subsystem  VariantControl=saturation_off
  Saturation on : Subsystem  VariantControl=saturation_on
  controlSignal : Outport

== system model_prawego_zbiornika/ADRC/ADRC controller/State feedback robust controller/Dead time/Dead time off ==
  In1 : Inport
  Out1 : Outport
  wires:
  In1/1 -> Out1/1

== system model_prawego_zbiornika/ADRC/ADRC controller/State feedback robust controller/Dead time/Dead time on ==
  In1 : Inport
  Product : Product
  Step : Step  Time=Time  SampleTime=0
  Out1 : Outport
  wires:
  Product/1 -> Out1/1
  Step/1 -> Product/2
  In1/1 -> Product/1

== system model_prawego_zbiornika/ADRC/ADRC controller/State feedback robust controller/Saturation/Saturation off ==
  In1 : Inport
  controlSignal : Outport
  wires:
  In1/1 -> controlSignal/1

== system model_prawego_zbiornika/ADRC/ADRC controller/State feedback robust controller/Saturation/Saturation on ==
  In1 : Inport
  Saturation : Saturate  UpperLimit=UpperLimit  LowerLimit=LowerLimit
  controlSignal : Outport
  wires:
  Saturation/1 -> controlSignal/1
  In1/1 -> Saturation/1

== matlab function model_prawego_zbiornika/ADRC/ADRC controller/State feedback robust controller/Extended state feedback robust controller ==
  data: inputGainParameter parameter; externalInputGainParameter input; controllerBandwidth parameter; controlSignal output size=1; estimatedExtendedState input; externalControllerBandwidth input; dynamicsOrder parameter
function controlSignal = fcn(inputGainParameter,...
        externalInputGainParameter,...
        controllerBandwidth,...
        estimatedExtendedState,...
        externalControllerBandwidth,...
        dynamicsOrder)
    
    usedInputGain = evaluateSource(inputGainParameter, externalInputGainParameter);
    usedControllerBandwidth = evaluateSource(controllerBandwidth, externalControllerBandwidth);
    K = calculateControllerGain(usedControllerBandwidth, dynamicsOrder);
    
    controlSignal = 1/usedInputGain * (estimatedExtendedState(end) +...
            K * estimatedExtendedState(1:end-1));
end

function output = evaluateSource(internal, external)
    if(external == 0)
        output = internal;
    else
        output = external;
    end
end

function controllerGain = calculateControllerGain(controllerBandwidth, dynamicsOrder)
    extendedControllerGain = poly(-controllerBandwidth * ones(1, dynamicsOrder));
    controllerGain = flip(extendedControllerGain(2:end));
end

== matlab function model_prawego_zbiornika/ADRC/ADRC controller/Linear extended state observer/Linear extended state observer ==
  data: previousEstimatedExtendedState input; controlError input; estimatedExtendedStateDerivative output; controlSignal input; dynamicsOrder parameter size=1; inputGainParameter parameter; externalInputGainParameter input; externalObserverBandwidth input; observerBandwidth parameter
function estimatedExtendedStateDerivative = fcn(previousEstimatedExtendedState,...
        controlError,...
        controlSignal,...
        dynamicsOrder,...
        inputGainParameter,...
        externalInputGainParameter,...
        externalObserverBandwidth,...
        observerBandwidth)
    
    usedInputGain = evaluateSource(inputGainParameter, externalInputGainParameter);
    usedObserverBandwidth = evaluateSource(observerBandwidth, externalObserverBandwidth);
    A = calculateObserverStateMatrix(dynamicsOrder);
    B = calculateObserverInputMatrix(usedInputGain, dynamicsOrder);
    L = calculateObserverGainVector(usedObserverBandwidth, dynamicsOrder);
    
    estimatedExtendedStateDerivative = A * previousEstimatedExtendedState +...
        B * controlSignal +...
        L * (controlError - previousEstimatedExtendedState(1));
end

function output = evaluateSource(internal, external)
    if(external == 0)
        output = internal;
    else
        output = external;
    end
end

function observerStateMatrix = calculateObserverStateMatrix(dynamicsOrder)
    observerStateMatrix = [zeros(dynamicsOrder,1), eye(dynamicsOrder);...
        zeros(1,dynamicsOrder+1)];
end

function observerInputMatrix = calculateObserverInputMatrix(inputGainParameter, dynamicsOrder)
    observerInputMatrix = [zeros(dynamicsOrder-1,1); -inputGainParameter; 0];
end

function observerGainVector = calculateObserverGainVector(observerBandwidth, dynamicsOrder)
    extendedGainVector = poly(-observerBandwidth * ones(1, dynamicsOrder+1))';
    observerGainVector = extendedGainVector(2:end);
end

== matlab function model_prawego_zbiornika/ADRC/ADRC controller/Observer output/Only estimated total disturbance/Last element of estimated extended state ==
  data: u input; y output
function y = last_element(u)
    y = u(end);
end

== matlab function model_prawego_zbiornika/ADRC/ADRC controller/Observer output/Only estimated control error/First element of estimated extended state ==
  data: u input; y output
function y = first_element(u)
    y = u(1);
end
